simulink model "master_task"  (Simulink 3.0)
libraries: mathlib x2, execlib x1, reglib x1, arclib x1

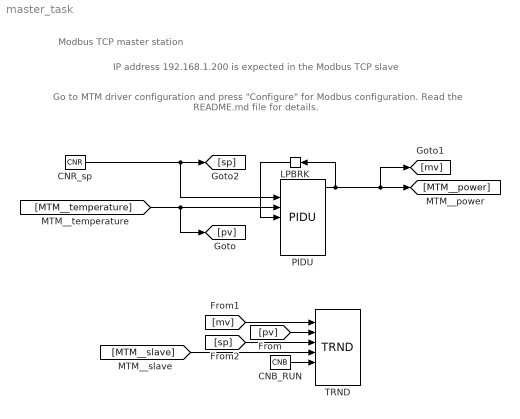
== system master_task ==
  note: Modbus TCP master station
  note: IP address 192.168.1.200 is expected in the Modbus TCP slave
  note: Go to MTM driver configuration and press "Configure" for Modbus configuration.
      |
      | Read the README.md file for details.
  CNB_RUN : mathlib/CNB  SystemSampleTime=-1  YCN=on
  CNR_sp : mathlib/CNR  ycn=75
  LPBRK : execlib/LPBRK  Orientation=left
  PIDU : reglib/PIDU  irtype=7: PID  RACT=off  k=0.281  ti=11.18  td=2.795  nd=10  b=0.7  c=0  tt=5.9  hilim=100  lolim=0  dz=0  icotype=1: Analog
  TRND : arclib/TRND  SystemSampleTime=-1  n=4  l=7200  btype=8: Double  ptype1=1: Store  ptype2=1: Store  ptype3=1: Store  ptype4=1: Store  pfac=1  afac=0  arc=0  id=1  Title=Trend Title  timesrc=1
  wires:
  CNB_RUN/1 -> TRND/5
  CNR_sp/1 -> [sp], PIDU/2
  [pv] -> TRND/2
  [mv] -> TRND/1
  [sp] -> TRND/3
  LPBRK/1 -> PIDU/4
  [MTM__slave] -> TRND/4
  [MTM__temperature] -> [pv], PIDU/3
  PIDU/1 -> LPBRK/1, [mv], [MTM__power]
